simulink model "PID_Test"  (R2023b)
settings: Solver=ode5  StartTime=0.0  StopTime=20  MaxStep=1  RelTol=1e-3  AbsTol=1e-3
libraries: simulink x4, slpidlib x1, softHIL x1
settings Model: Creator=mkottman  LastModifiedBy=Alex
settings SolverCC: AutoScaleAbsTol=off  AlgebraicLoopSolver=TrustRegion
settings DataIOCC: SaveFormat=Array  SignalLoggingSaveFormat=ModelDataLogs  SaveOutput=off  SaveTime=off  ReturnWorkspaceOutputs=off
settings OptimizationCC: BooleanDataType=off  ExpressionDepthLimit=2147483647  InitFltsAndDblsToZero=on  LifeSpan=inf
settings DebuggingCC: SaveWithParameterizedLinksMsg=none  UnderspecifiedInitializationDetection=Classic  MergeDetectMultiDrivingBlocksExec=none  SignalResolutionControl=TryResolveAllWithWarning  MultiTaskDSMMsg=warning  MultiTaskCondExecSysMsg=none  FcnCallInpInsideContextMsg=warning  UnconnectedInputMsg=warning  UnconnectedOutputMsg=warning  UnconnectedLineMsg=warning  StateNameClashWarn=warning  SFUnexpectedBacktrackingDiag=warning  SFNoUnconditionalDefaultTransitionDiag=warning  SFExecutionAtInitializationDiag=none  ArithmeticOperatorsInVariantConditions=warning
settings HardwareCC: ProdBitPerPointer=32  ProdBitPerSizeT=32  ProdBitPerPtrDiffT=32  ProdLargestAtomicFloat=None  ProdIntDivRoundTo=Undefined  ProdEndianess=Unspecified  ProdWordSize=32  ProdHWDeviceType=32-bit Generic  TargetUnknown=on
settings ModelReferenceCC: EnableRefExpFcnMdlSchedulingChecks=on  PropagateSignalLabelsOutOfModel=off
settings SFSimCC: SimUseLocalCustomCode=off  CustomCodeUndefinedFunction=UseInterfaceOnly
settings RTWCC: TemplateMakefile=grt_vc.tmf  RTWUseLocalCustomCode=off
settings CodeAppCC: StateflowObjectComments=on
settings GRTTargetCC: TargetFcnLib=ansi_tfl_tmw.mat  TargetLangStandard=C89/C90 (ANSI)  CombineOutputUpdateFcns=off  GRTInterface=on
settings ConfigComp: CovMetricSettings=dw  CovSaveCumulativeToWorkspaceVar=on  CovSaveSingleToWorkspaceVar=on  CovExternalEMLEnable=off

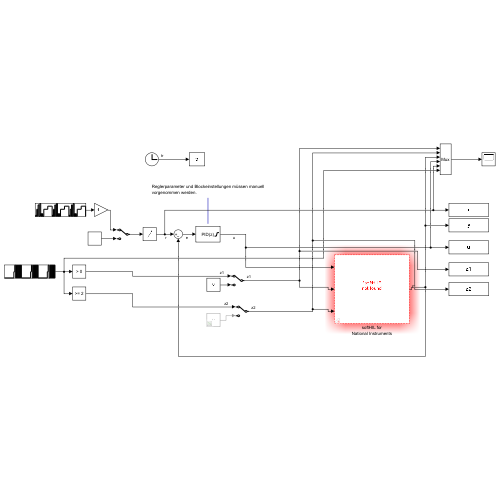
[thumbnail: Simulink's stored preview of the top-level diagram]
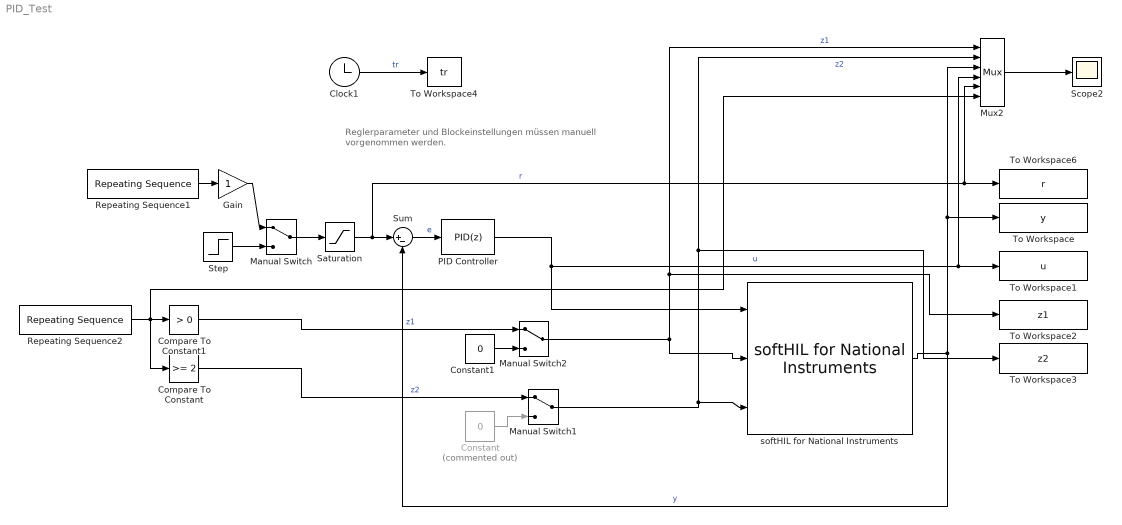
== system PID_Test ==
  note: Reglerparameter und Blockeinstellungen müssen manuell
      | vorgenommen werden.
  Clock1 : Clock
  Compare To Constant : simulink/Logic and Bit Operations/Compare To Constant  relop=>=  const=2  OutDataTypeStr=boolean
  Compare To Constant1 : simulink/Logic and Bit Operations/Compare To Constant  relop=>  const=0  OutDataTypeStr=boolean
  Constant : Constant  Commented=on  Value=0  SampleTime=0.01
  Constant1 : Constant  Value=0  SampleTime=0.01
  Gain : Gain
  Manual Switch : ManualSwitch
  Manual Switch1 : ManualSwitch
  Manual Switch2 : ManualSwitch
  Mux2 : Mux  Inputs=6
  PID Controller : slpidlib/PID Controller  Controller=PID  Form=Parallel  TimeDomain=Discrete-time  UseExternalTs=off  SampleTime=0.01  IntegratorMethod=Forward Euler  FilterMethod=Forward Euler  ControllerParametersSource=internal  P=6.124  I=84.536  UseKiTs=off  D=-0.487648  N=0.622535  UseFilter=on  TunerSelectOption=Transfer Function Based (PID Tuner App)  InitialConditionSource=internal  InitialConditionForIntegrator=0  InitialConditionForFilter=0  DifferentiatorICPrevScaledInput=0  ExternalReset=none  TrackingMode=off  Kt=1  LimitOutput=on  SatLimitsSource=internal  UpperSaturationLimit=10  LowerSaturationLimit=0  LinearizeAsGain=on  AntiWindupMode=clamping  Kb=1  LimitIntegrator=on  UpperIntegratorSaturationLimit=10  LowerIntegratorSaturationLimit=-10  POutMin=[]  POutMax=[]  IOutMin=[]  IOutMax=[]  DOutMin=[]  DOutMax=[]  NOutMin=[]  NOutMax=[]  SumOutMin=[]  SumOutMax=[]  SaturationOutMin=[]  SaturationOutMax=[]  PParamMin=[]  PParamMax=[]  IParamMin=[]  IParamMax=[]  DParamMin=[]  DParamMax=[]  NParamMin=[]  NParamMax=[]  KbParamMin=[]  KbParamMax=[]  KtParamMin=[]  KtParamMax=[]  KbOutMin=[]  KbOutMax=[]  KtOutMin=[]  KtOutMax=[]  IntegratorOutMin=[]  IntegratorOutMax=[]  FilterOutMin=[]  FilterOutMax=[]  SumI1OutMin=[]  SumI1OutMax=[]  SumI2OutMin=[]  SumI2OutMax=[]  SumI3OutMin=[]  SumI3OutMax=[]  SumI4OutMin=[]  SumI4OutMax=[]  SumDOutMin=[]  SumDOutMax=[]  DifferentiatorOutMin=[]  DifferentiatorOutMax=[]  FilterDiffOutCoefMin=[]  FilterDiffOutCoefMax=[]  ReciprocalOutMin=[]  ReciprocalOutMax=[]  SumDenOutMin=[]  SumDenOutMax=[]  SumNumOutMin=[]  SumNumOutMax=[]  DivideOutMin=[]  DivideOutMax=[]  UdiffTsProdOutMin=[]  UdiffTsProdOutMax=[]  NTsProdOutMin=[]  NTsProdOutMax=[]  UintegralTsProdOutMin=[]  UintegralTsProdOutMax=[]  UngainTsProdOutMin=[]  UngainTsProdOutMax=[]  ClampingZeroOutDataTypeStr=Inherit: Inherit via back propagation  ClampingZeroOutMin=[]  ClampingZeroOutMax=[]  FilterDenConstantOutDataTypeStr=Inherit: Inherit via back propagation  FilterDenConstantOutMin=[]  FilterDenConstantOutMax=[]  PCopyOutDataTypeStr=Inherit: Inherit via back propagation  PCopyOutMin=[]  PCopyOutMax=[]  NCopyOutDataTypeStr=Inherit: Inherit via back propagation  NCopyOutMin=[]  NCopyOutMax=[]  IntegratorContinuousStateAttributes=''  IntegratorStateMustResolveToSignalObject=off  IntegratorRTWStateStorageClass=Auto  FilterContinuousStateAttributes=''  FilterStateMustResolveToSignalObject=off  FilterRTWStateStorageClass=Auto  ParallelPVariant=InternalParameters  IdealPVariant=Disabled  IVariant=InternalParameters  DVariant=InternalParameters  IntegratorVariant=Discrete  SatVariant=Enabled  AWVariant=DiscClampingParallel  PCopyVariant=Disabled  TRVariant=Disabled  FdbkBlocksVariant=Forward  IdealPFdbkVariant=Disabled  SatFdbkVariant=Disabled  DerivativeFilterVariant=ForwardEulerFilter  NVariant=InternalParameters  NCopyVariant=Disabled  FilterICVariant=InternalICsFilter  IntegratorICVariant=InternalICs  ExternalResetVariant=Disabled  TRSumVariant=Passthrough  SumFdbkVariant=Disabled  SumVariant=Sum_PID  TsampFilterVariant=InternalTs  TsampNgainVariant=Passthrough  TsampIntegralVariant=Disabled_SignalSpec  ExternalSaturationOutDataTypeStr=Inherit: Same as second input
  Repeating Sequence1 : simulink/Sources/Repeating Sequence  rep_seq_t=[0.000000 0.490000 0.500000 0.990000 1.000000 1.490000 1.500000 2.490000 2.500000 3.490000 3.500000 4.490000 4.500000 5.490000 5.500000 6.240000 6.250000 6.490000 6.500000 6.990000 7.000000 7.490000 7.500000 7.990000 8.000000 8.490000 8.500000 8.990000 9.000000 9.990000 10.000000 14.990000 15.000000 19.990000 20.500000 ]  rep_seq_y=[0.000000 0.000000 1.000000 1.000000 0.000000 0.000000 5.000000 5.000000 0.000000 0.000000 8.000000 8.000000 0.000000 0.000000 9.000000 9.000000 0.000000 0.000000 2.000000 2.000000 0.000000 0.000000 2.000000 2.000000 0.000000 0.000000 2.000000 2.000000 0.000000 0.000000 5.000000 5.000000 7.000000 7.000000 7.000000 ]
  Repeating Sequence2 : simulink/Sources/Repeating Sequence  rep_seq_t=[0.000000 10.990000 11.000000 11.990000 12.000000 12.990000 13.000000 13.990000 14.000000 14.490000 14.500000 14.990000 15.000000 15.490000 15.500000 15.990000 16.000000 16.490000 16.500000 16.990000 17.000000 17.490000 17.500000 17.990000 18.000000 18.490000 18.500000 18.990000 19.000000 19.490000 19.500000 ]  rep_seq_y=[0.000000 0.000000 1.000000 1.000000 2.000000 2.000000 0.000000 0.000000 2.000000 2.000000 0.000000 0.000000 2.000000 2.000000 0.000000 0.000000 2.000000 2.000000 0.000000 0.000000 2.000000 2.000000 0.000000 0.000000 2.000000 2.000000 0.000000 0.000000 2.000000 2.000000 0.000000 ]
  Saturation : Saturate  UpperLimit=10  LowerLimit=0
  Scope2 : Scope
  Step : Step  After=5  SampleTime=0.01
  Sum : Sum  Inputs=|+-
  To Workspace : ToWorkspace  VariableName=y  SaveFormat=Timeseries  SampleTime=0.01
  To Workspace1 : ToWorkspace  VariableName=u  SaveFormat=Timeseries  SampleTime=0.01
  To Workspace2 : ToWorkspace  VariableName=z1  SaveFormat=Timeseries  SampleTime=0.01
  To Workspace3 : ToWorkspace  VariableName=z2  SaveFormat=Timeseries  SampleTime=0.01
  To Workspace4 : ToWorkspace  VariableName=tr  SampleTime=5/1000
  To Workspace6 : ToWorkspace  VariableName=r  SaveFormat=Timeseries  SampleTime=0.01
  softHIL for National Instruments : softHIL/softHIL for National Instruments  nAIn=1  nAOut=1  nDIn=0  nDOut=2  Sampletime=0.01  Servername=getservername  ServerOL=off  ClientOL=off  Delay=off
  wires:
  Clock1/1 -> To Workspace4/1  "tr"
  Mux2/1 -> Scope2/1
  softHIL for National Instruments/1 -> Mux2/3, To Workspace/1, Sum/2  "y"
  Manual Switch2/1 -> softHIL for National Instruments/2, Mux2/1, To Workspace2/1  "z1"
  Manual Switch1/1 -> Mux2/2, To Workspace3/1, softHIL for National Instruments/3  "z2"
  Step/1 -> Manual Switch/2
  Sum/1 -> PID Controller/1  "e"
  PID Controller/1 -> To Workspace1/1, Mux2/4, softHIL for National Instruments/1  "u"
  Manual Switch/1 -> Saturation/1
  Repeating Sequence1/1 -> Gain/1
  Saturation/1 -> Mux2/5, To Workspace6/1, Sum/1  "r"
  Compare To Constant/1 -> Manual Switch1/1  "z2"
  Constant/1 -> Manual Switch1/2
  Compare To Constant1/1 -> Manual Switch2/1  "z1"
  Constant1/1 -> Manual Switch2/2
  Repeating Sequence2/1 -> Mux2/6, Compare To Constant1/1, Compare To Constant/1
  Gain/1 -> Manual Switch/1
